simulink model "sl_partitioned"  (R2016a)
settings: Solver=ode45  StartTime=0.0  StopTime=160  RelTol=1e-3
InitFcn:
  | cam = CentralCamera('default')
undefined symbols (not defined in the file or in its folder): angdiff, mkgrid, mpq_poly, transl, trotz
libraries: roblocks x6
settings Model: ExtModeTrigMode=oneshot  ExtModeArmWhenConnect=off  Creator=pic  LastModifiedBy=corkep
settings DataIOCC: SaveFormat=Structure  SignalLoggingSaveFormat=ModelDataLogs  ReturnWorkspaceOutputs=on
settings OptimizationCC: BlockReduction=off  BooleanDataType=off  ExpressionDepthLimit=2147483647  InitFltsAndDblsToZero=on
settings DebuggingCC: SaveWithParameterizedLinksMsg=none  UnderspecifiedInitializationDetection=Classic  MergeDetectMultiDrivingBlocksExec=none  SignalResolutionControl=TryResolveAllWithWarning  MultiTaskDSMMsg=warning  MultiTaskCondExecSysMsg=none  FcnCallInpInsideContextMsg=UseLocalSettings  AllowSymbolicDim=off  StateNameClashWarn=warning
settings HardwareCC: ProdBitPerPointer=32  ProdLargestAtomicFloat=None  ProdIntDivRoundTo=Undefined  ProdEndianess=Unspecified  ProdWordSize=32  ProdHWDeviceType=32-bit Generic  TargetUnknown=on
settings ModelReferenceCC: PropagateSignalLabelsOutOfModel=off
settings GRTTargetCC: ModelReferenceCompliant=off  CompOptLevelCompliant=off  CombineOutputUpdateFcns=off  MatFileLogging=off  GRTInterface=on
settings ConfigComp: CovModelRefEnable=Off  CovSFcnEnable=off

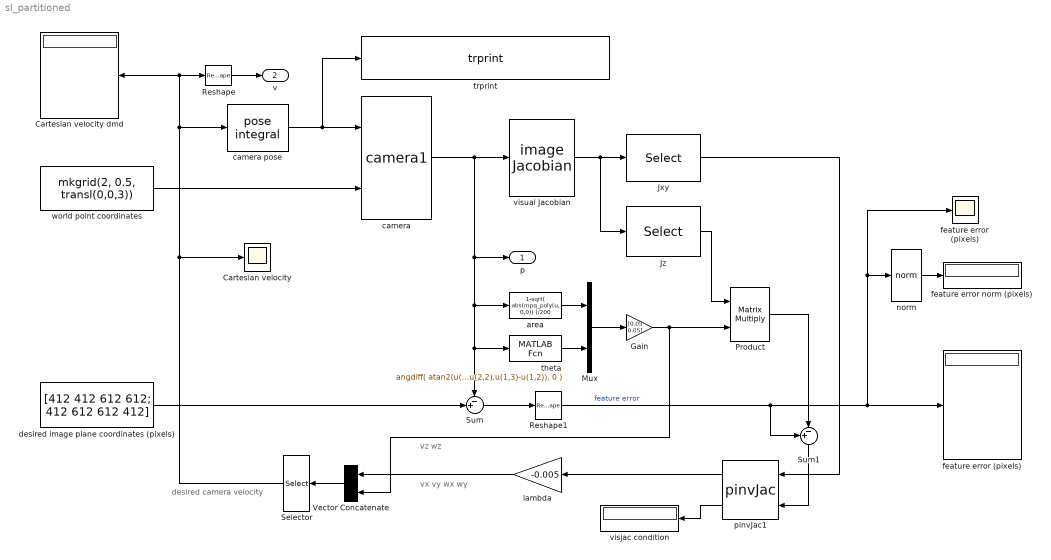
== system sl_partitioned ==
  note: vz wz
  note: vx vy wx wy
  note: desired camera velocity
  Cartesian velocity : Scope
  Cartesian velocity dmd : Display
      settings: Format=bank
  Gain : Gain  Gain=[0.05 0.05]
  Jxy : Selector  NumberOfDimensions=2  InputPortWidth=3  IndexOptions=Select all,Index vector (dialog)  Indices=[1 3],[1 2 4 5]  OutputSizes=1,1
  Jz : Selector  NumberOfDimensions=2  InputPortWidth=3  IndexOptions=Select all,Index vector (dialog)  Indices=[1 3],[3 6]  OutputSizes=1,1
  Mux : Mux  Inputs=2
  Product : Product  Multiplication=Matrix(*)  RndMeth=Zero
  Reshape : Reshape  OutputDimensions=6
  Reshape1 : Reshape  OutputDimensions=6
  Selector : Selector  InputPortWidth=6  IndexOptions=Index vector (dialog)  Indices=[1 2 5 3 4 6]  OutputSizes=1
  Sum : Sum  Inputs=-+|  SaturateOnIntegerOverflow=on  InputSameDT=on  OutDataTypeStr=Inherit: Same as first input
  Sum1 : Sum  Inputs=+-|
  Vector Concatenate : Concatenate  ConcatenateDimension=2
  area : MATLABFcn  MATLABFcn=1-sqrt( abs(mpq_poly(u, 0,0)) )/200
  camera : roblocks/Vision/camera1  cam=cam
  camera pose : roblocks/Toolbox/pose integral  T0=transl(0,0,1)*trotz(1.5)  dt=0.02
  desired image plane coordinates (pixels) : Constant  Value=[412 412 612 612; 412 612 612 412]  VectorParams1D=off
  feature error norm (pixels) : Display
  feature error (pixels) : Display
      settings: Format=bank
  "feature error (pixels) " : Scope
  lambda : Gain  Gain=-0.005  SaturateOnIntegerOverflow=on  OutDataTypeStr=Inherit: Same as input  ParamDataTypeStr=Inherit: Same as input
  norm : roblocks/Toolbox/norm  SystemSampleTime=-1
  pinvJac1 : roblocks/Toolbox/pinvJac
  theta : MATLABFcn  MATLABFcn=angdiff( atan2(u(2,3)-u(2,2),u(1,3)-u(1,2)), 0 )
  trprint : roblocks/Toolbox/trprint  options={}
      link override S-Function: Parameters=options
  visjac condition : Display
  visual Jacobian : roblocks/Vision/image Jacobian  cam=cam  z=3
  world point coordinates : Constant  Value=mkgrid(2, 0.5, transl(0,0,3))  VectorParams1D=off
  p : Outport
  v : Outport  Port=2
  wires:
  Sum/1 -> Reshape1/1
  desired image plane coordinates (pixels)/1 -> Sum/2
  Reshape1/1 -> Sum1/1, feature error (pixels)/1, "feature error (pixels) "/1, norm/1  "feature error"
  pinvJac1/1 -> lambda/1
  camera pose/1 -> trprint/1, camera/1
  Reshape/1 -> v/1
  camera/1 -> theta/1, Sum/1, area/1, p/1, visual Jacobian/1
  world point coordinates/1 -> camera/2
  norm/1 -> feature error norm (pixels)/1
  Jxy/1 -> pinvJac1/1
  Selector/1 -> Reshape/1, Cartesian velocity dmd/1, camera pose/1, Cartesian velocity/1
  Vector Concatenate/1 -> Selector/1
  lambda/1 -> Vector Concatenate/1
  theta/1 -> Mux/2
  Mux/1 -> Gain/1
  Gain/1 -> Vector Concatenate/2, Product/2
  area/1 -> Mux/1
  visual Jacobian/1 -> Jz/1, Jxy/1
  Jz/1 -> Product/1
  Sum1/1 -> pinvJac1/2
  Product/1 -> Sum1/2
  pinvJac1/2 -> visjac condition/1
